simulink model "srotut2"  (Simulink 6.0)
settings: Solver=ode45  SolverMode=SingleTasking  StartTime=0  StopTime=1  RelTol=1e-4  AbsTol=1e-6
PreLoadFcn:
  | load srotut2_dat
undefined symbols (not defined in the file or in its folder): C2, K, Qmax
libraries: hydlib x2, srolib x2
settings Model: CovMetricSettings=d  Creator=monteiro  LastModifiedBy=lparsons  ExtModeTrigMode=oneshot  ExtModeArmWhenConnect=off  ExtModeAutoUpdateStatusClock=off
settings DataIOCC: LimitDataPoints=off  SaveState=on  SignalLoggingName=logsOut
settings OptimizationCC: BlockReduction=off  BooleanDataType=off
settings DebuggingCC: AlgebraicLoopMsg=none  CheckExecutionContextPreStartOutputMsg=on  CheckExecutionContextRuntimeOutputMsg=on  SolverPrmCheckMsg=none  IntegerOverflowMsg=none
settings HardwareCC: TargetUnknown=on
settings SFSimCC: SFSimApplyToAllLibs=on  SFSimBuildMode=Incremental

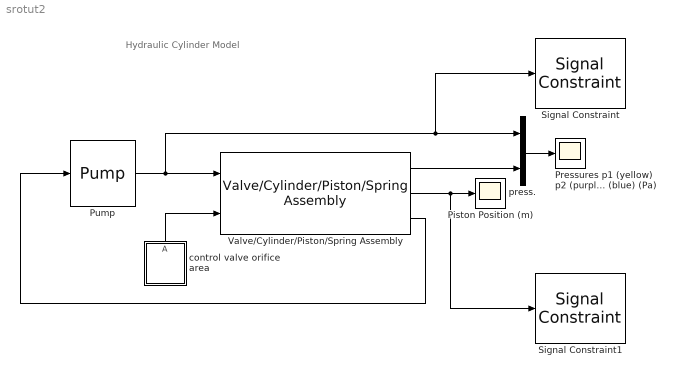
== system srotut2 ==
  note: Hydraulic Cylinder Model
  Piston Position (m) : Scope
      settings: TickLabels=on  TimeRange=0.1  YMin=0  YMax=0.04  DataFormat=Array
  Pressures p1 (yellow) p2 (purple) p3 (blue) (Pa) : Scope
      settings: TickLabels=on  TimeRange=0.1  YMin=0  YMax=2e+006  DataFormat=Array
  Pump : hydlib/Pump  t=linspace(0,2,1000)  Qpump=Qmax*ones(1,1000)  p10=Qmax/C2*2  C2=C2
  Signal Constraint : srolib/Signal Constraint  DialogPosition=[0.0512152777777778 0.056712962962963 0.450520833333333 0.310185185185185]  SaveIn=workspace  LogID=SRO_DataLog_1
  Signal Constraint1 : srolib/Signal Constraint  DialogPosition=[0.508680555555556 0.056712962962963 0.450520833333333 0.310185185185185]  SaveIn=workspace  LogID=SRO_DataLog_2
  Valve/Cylinder/Piston/Spring Assembly : hydlib/Valve//Cylinder//Piston//Spring Assembly  K=K  C1=C1  Ac=Ac  Cd=Cd  rho=rho  V30=V30  beta=Beta
  control valve orifice area : Subsystem  Orientation=up  PropExecContextAcrossSSBoundary=on
      mask Type: Ramp
      mask Display: plot(0,0,100,100,[98,0],[96,0])
  press. : Mux  Inputs=2
  wires:
  control valve orifice area/1(A) -> Valve/Cylinder/Piston/Spring Assembly/2
  Pump/1 -> Valve/Cylinder/Piston/Spring Assembly/1, press./1, Signal Constraint/1
  press./1 -> Pressures p1 (yellow) p2 (purple) p3 (blue) (Pa)/1
  Valve/Cylinder/Piston/Spring Assembly/2 -> Piston Position (m)/1, Signal Constraint1/1
  Valve/Cylinder/Piston/Spring Assembly/1 -> press./2
  Valve/Cylinder/Piston/Spring Assembly/3 -> Pump/1

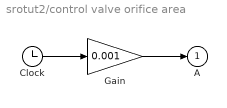
== system srotut2/control valve orifice area ==
  Clock : Clock
      settings: Decimation=10
  Gain : Gain  Gain=0.001  SaturateOnIntegerOverflow=on
  A : Outport  InitialOutput=0
  wires:
  Gain/1 -> A/1
  Clock/1 -> Gain/1
